simulink model "ADC"  (R2015a)
settings: Solver=ode4  StartTime=t0  StopTime=tf  FixedStep=dt  RelTol=1e-6
InitFcn:
  | sat_model_init
undefined symbols (not defined in the file or in its folder): Continuous, Time
libraries: simulink x1, ctrlSharedLib x1, dspmathops x1
settings Model: SimulationMode=external  Creator=Josue  LastModifiedBy=jbparham
settings DataIOCC: SignalLoggingSaveFormat=ModelDataLogs  SaveOutput=off  SaveState=on  SaveTime=off
settings OptimizationCC: ExpressionDepthLimit=2147483647  EfficientMapNaN2IntZero=off  OptimizeModelRefInitCode=on  LifeSpan=Inf
settings DebuggingCC: ReadBeforeWriteMsg=DisableAll  WriteAfterWriteMsg=DisableAll  WriteAfterReadMsg=DisableAll  UnderspecifiedInitializationDetection=Classic  MergeDetectMultiDrivingBlocksExec=none  SolverPrmCheckMsg=warning  MultiTaskDSMMsg=warning  MultiTaskCondExecSysMsg=none  FcnCallInpInsideContextMsg=UseLocalSettings  StateNameClashWarn=warning
settings HardwareCC: TargetBitPerLong=64  TargetBitPerPointer=64  TargetLongLongMode=on  TargetIntDivRoundTo=Zero  TargetEndianess=LittleEndian  TargetWordSize=64  TargetHWDeviceType=MATLAB Host  ProdEqTarget=off
settings ModelReferenceCC: ModelReferenceNumInstancesAllowed=Single
settings SFSimCC: SimParseCustomCode=off
settings RTWCC: SystemTargetFile=ert.tlc  TemplateMakefile=ert_default_tmf  Description=Embedded Coder  GenerateReport=on  IncludeHyperlinkInReport=on  LaunchReport=on
settings CodeAppCC: IgnoreCustomStorageClasses=off  MaxIdLength=128
settings ERTTargetCC: ParMdlRefBuildCompliant=on  CompOptLevelCompliant=on  ConcurrentExecutionCompliant=on  ERTFirstTimeCompliant=on  ModelStepFunctionPrototypeControlCompliant=on  CPPClassGenCompliant=on  InlinedParameterPlacement=Hierarchical  ERTCustomFileTemplate=example_file_process.tlc

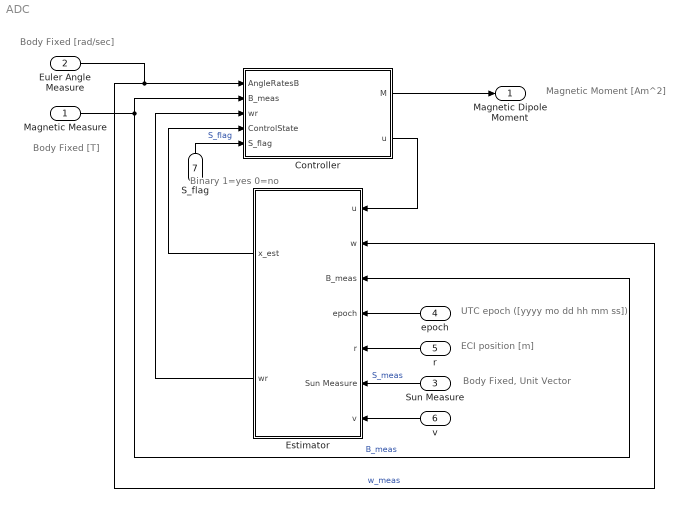
== system ADC ==
  note: Magnetic Moment [Am^2]
  note: Binary 1=yes 0=no
  note: ECI position [m]
  note: UTC epoch ([yyyy mo dd hh mm ss])
  note: Body Fixed, Unit Vector
  note: Body Fixed [rad/sec]
  note: Body Fixed [T]
  Magnetic Measure : Inport  OutDataTypeStr=double  PortDimensions=3  SampleTime=0
  Euler Angle Measure : Inport  Port=2  OutDataTypeStr=double  PortDimensions=3  SampleTime=0
  Sun Measure : Inport  Port=3  OutDataTypeStr=double  PortDimensions=3  SampleTime=0
  epoch : Inport  Port=4  OutDataTypeStr=double  PortDimensions=6
  r : Inport  Port=5  OutDataTypeStr=double  PortDimensions=3  SampleTime=0
  "v " : Inport  Port=6  OutDataTypeStr=double  PortDimensions=3  SampleTime=0
  S_flag : Inport  Port=7  OutDataTypeStr=double  PortDimensions=1  SampleTime=0
  Controller : Subsystem
  Estimator : Subsystem
  Magnetic Dipole Moment : Outport  OutDataTypeStr=double  PortDimensions=3  SampleTime=0
  wires:
  Magnetic Measure/1 -> Estimator/3(B_meas), Controller/2(B_meas)  "B_meas"
  Euler Angle Measure/1 -> Controller/1(AngleRatesB), Estimator/2(w)  "w_meas"
  Controller/1(M) -> Magnetic Dipole Moment/1
  Controller/2(u) -> Estimator/1(u)
  epoch/1 -> Estimator/4(epoch)
  r/1 -> Estimator/5(r)
  Sun Measure/1 -> Estimator/6(Sun Measure)  "S_meas"
  "v "/1 -> Estimator/7("v ")
  Estimator/1(x_est) -> Controller/4(ControlState)
  S_flag/1 -> Controller/5(S_flag)  "S_flag"
  Estimator/2(wr) -> Controller/3(wr)

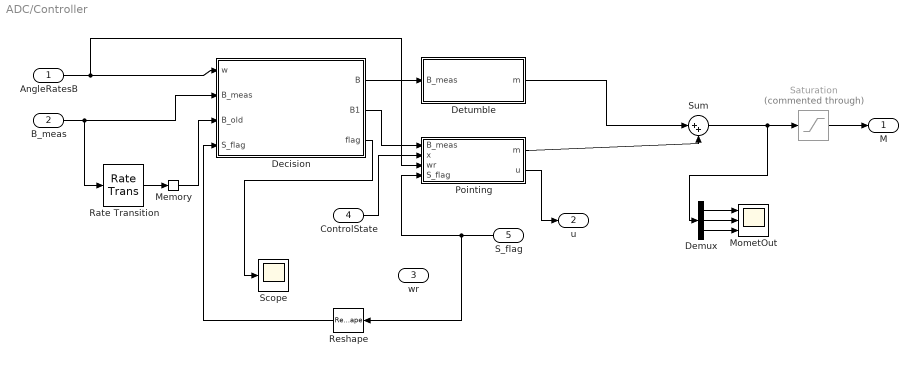
== system ADC/Controller ==
  AngleRatesB : Inport
  B_meas : Inport  Port=2
  wr : Inport  Port=3
  ControlState : Inport  Port=4
  S_flag : Inport  Port=5
  Decision : MATLAB Function  TreatAsAtomicUnit=on
  Demux : Demux  Outputs=3
  "Detumble " : Subsystem
  Memory : Memory  InheritSampleTime=on
  MometOut : Scope  NumInputPorts=3
      settings: YMin=-0.008~-0.015~-0.008  YMax=0.004~0.0175~0.002
  Pointing : Subsystem
  Rate Transition : RateTransition  OutPortSampleTime=.1
  Reshape : Reshape  OutputDimensionality=Customize
  Saturation : Saturate  Commented=through  UpperLimit=1  LowerLimit=-1
  Scope : Scope
      settings: YMin=0.95  YMax=1.05  SaveName=ScopeData5
  Sum : Sum  Inputs=|++
  M : Outport
  u : Outport  Port=2
  wires:
  Rate Transition/1 -> Memory/1
  S_flag/1 -> Reshape/1, Pointing/4(S_flag)
  Reshape/1 -> Decision/4(S_flag)
  B_meas/1 -> Decision/2(B_meas), Rate Transition/1
  Pointing/1(m) -> Sum/2
  Saturation/1 -> M/1
  Decision/3(flag) -> Scope/1
  Memory/1 -> Decision/3(B_old)
  Demux/3 -> MometOut/3
  Demux/2 -> MometOut/2
  Demux/1 -> MometOut/1
  Pointing/2(u) -> u/1
  ControlState/1 -> Pointing/2(x)
  Decision/2(B1) -> Pointing/1(B_meas)
  Decision/1(B) -> "Detumble "/1("B_meas ")
  "Detumble "/1(m) -> Sum/1
  Sum/1 -> Saturation/1, Demux/1
  AngleRatesB/1 -> Decision/1(w), Pointing/3(wr)

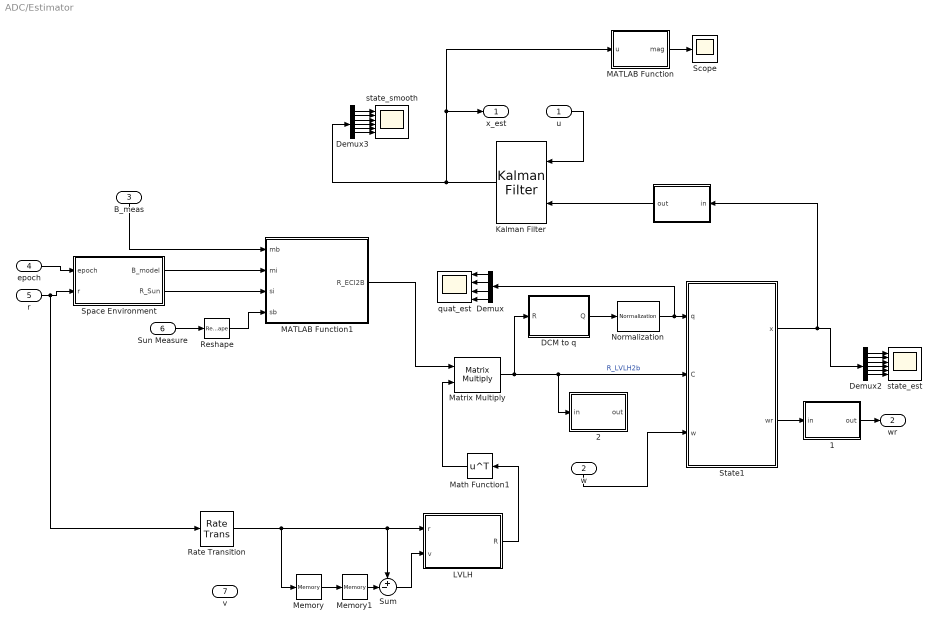
== system ADC/Estimator ==
  u : Inport
  w : Inport  Port=2
  B_meas : Inport  Port=3
  epoch : Inport  Port=4
  r : Inport  Port=5
  Sun Measure : Inport  Port=6
  "v " : Inport  Port=7
  " " : MATLAB Function  TreatAsAtomicUnit=on
  " 1" : MATLAB Function  TreatAsAtomicUnit=on
  " 2" : MATLAB Function  TreatAsAtomicUnit=on
  " LVLH " : MATLAB Function  TreatAsAtomicUnit=on
  DCM to q : MATLAB Function  TreatAsAtomicUnit=on
  Demux : Demux
  Demux2 : Demux  Outputs=6
  Demux3 : Demux  Outputs=6
  Kalman Filter : ctrlSharedLib/Kalman Filter  TimeDomain=Continuous-Time  UseCurrentEstimator=on  ModelSource=Individual A, B, C, D matrices  ModelSourceVariable=ss(0.95,1,1,0,1)  A=[0,0,0,1,0,0;0,0,0,0,1,0;0,0,0,0,0,1;3.26658658709613e-06,0,0,0,0,0.00184463935812897;0,2.93992792838652e-06,0,0,0,0;0,0,-3.49991420046014e-07,-0.000790559724912417,0,0]  B=[zeros(3);eye(3)]  C=eye(6)  D=0  NumberOfStates=1  NumberOfInputs=1  NumberOfOutputs=1  InitialEstimateSource=Dialog  X0=zeros(6,1)  P0=10  UseK=off  UseGH=off  NumberOfProcessNoiseInputs=1  G=1  TimeInvariantG=on  H=0  TimeInvariantH=on  Q=1  TimeInvariantQ=on  R=[.5*eye(3),zeros(3);zeros(3),0.005*eye(3)]  TimeInvariantR=on  N=0  TimeInvariantN=on  AddInputPort=on  AddEnablePort=off  ExternalReset=none  OutputEstimatedY=off  OutputP=off  Ts=.1
  MATLAB Function : MATLAB Function  TreatAsAtomicUnit=on
  MATLAB Function1 : MATLAB Function  TreatAsAtomicUnit=on
  Math Function1 : Math  Operator=transpose  SaturateOnIntegerOverflow=on
  Matrix Multiply : Product  Multiplication=Matrix(*)
  Memory : Memory
  Memory1 : Memory
  Normalization : dspmathops/Normalization  NormType=Squared 2-norm  Bias=1e-10  NormOver=Each column  ColComp=off  Dimension=1  outputDataTypeStr=Inherit: Same as product output  outputLastDataTypeStr=Inherit: Same as product output  outputMin=[]  outputMax=[]  accumDataTypeStr=Inherit: Same as product output  accumLastDataTypeStr=Inherit: Same as product output  roundingMode=Floor  overflowMode=off
  Rate Transition : RateTransition  OutPortSampleTime=.1
  Reshape : Reshape  OutputDimensionality=Customize  OutputDimensions=[3,1]
  Scope : Scope
      settings: YMin=5.55112e-17  YMax=1.4  SaveName=ScopeData3
  Space Environment : Subsystem
  State1 : MATLAB Function  TreatAsAtomicUnit=on
  Sum : Sum  Inputs=+-|
  quat_est : Scope  NumInputPorts=4
      settings: ShowLegends=on  YMin=-1.24924~-1.24976~-1.2264~-0.115999  YMax=1.24823~1.24976~1.22612~1.04399  SaveName=quat_est  DataFormat=Structure
  state_est : Scope  NumInputPorts=6
      settings: ShowLegends=on  YMin=-1.23534~-1.22576~-1.24248~-0.102409~-0.112864~-0.0966162  YMax=1.24677~1.22585~1.24228~0.115625~0.0969559~0.105  SaveName=quat_est1  DataFormat=Structure
  state_smooth : Scope  NumInputPorts=6
      settings: ShowLegends=on  YMin=-1~-1~-1~-0.075~-0.1~-0.075  YMax=1~1~1~0.1~0.075~0.1  SaveName=ScopeData4  DataFormat=Structure
  x_est : Outport
  wr : Outport  Port=2
  wires:
  Rate Transition/1 -> Memory/1, Sum/1, " LVLH "/1(r)
  Sum/1 -> " LVLH "/2(v)
  Memory1/1 -> Sum/2
  Memory/1 -> Memory1/1
  Reshape/1 -> MATLAB Function1/4(sb)
  Sun Measure/1 -> Reshape/1
  Kalman Filter/1 -> x_est/1, MATLAB Function/1(u), Demux3/1
  " "/1(out) -> Kalman Filter/2
  u/1 -> Kalman Filter/1
  Demux3/6 -> state_smooth/6
  Demux3/5 -> state_smooth/5
  Demux3/3 -> state_smooth/3
  Demux3/4 -> state_smooth/4
  Demux3/2 -> state_smooth/2
  Demux3/1 -> state_smooth/1
  " 1"/1(out) -> wr/1
  State1/2(wr) -> " 1"/1(in)
  Demux2/6 -> state_est/6
  Demux2/5 -> state_est/5
  Demux2/3 -> state_est/3
  Demux2/4 -> state_est/4
  Demux2/2 -> state_est/2
  Demux2/1 -> state_est/1
  State1/1(x) -> Demux2/1, " "/1(in)
  B_meas/1 -> MATLAB Function1/1(mb)
  w/1 -> State1/3(w)
  MATLAB Function1/1(R_ECI2B) -> Matrix Multiply/1
  Space Environment/1(B_model) -> MATLAB Function1/2(mi)
  MATLAB Function/1(mag) -> Scope/1
  Normalization/1 -> State1/1(q), Demux/1
  Space Environment/2(R_Sun) -> MATLAB Function1/3(si)
  Demux/3 -> quat_est/3
  Matrix Multiply/1 -> DCM to q/1(R), State1/2(C), " 2"/1(in)  "R_LVLH2b"
  Demux/4 -> quat_est/4
  Demux/2 -> quat_est/2
  epoch/1 -> Space Environment/1(epoch)
  r/1 -> Rate Transition/1, Space Environment/2(r)
  DCM to q/1(Q) -> Normalization/1
  Demux/1 -> quat_est/1
  Math Function1/1 -> Matrix Multiply/2
  " LVLH "/1(R) -> Math Function1/1

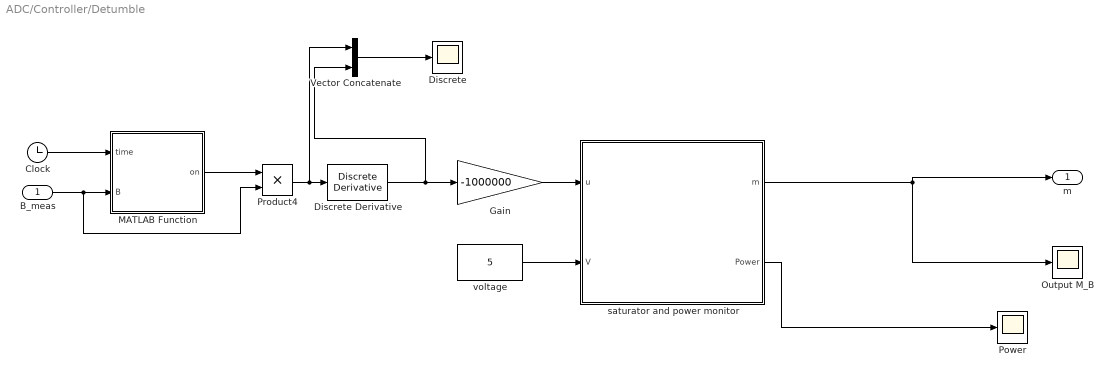
== system ADC/Controller/Detumble  ==
  "B_meas " : Inport
  Clock : Clock
  "Discrete " : Scope
      settings: ShowLegends=on  TimeRange=0.0243621865078012  YMin=-5.004965470144639e-05  YMax=3.166418994305964e-05  SaveName=ScopeData2
  Discrete Derivative : simulink/Discrete/Discrete Derivative  gainval=1.0  ICPrevScaledInput=0  InputProcessing=Inherited  OutMin=[]  OutMax=[]  OutDataType=fixdt(1, 16)  OutScaling=2^-10  DoSatur=off
  Gain : Gain  Gain=-1000000
  MATLAB Function : MATLAB Function  TreatAsAtomicUnit=on
  Output M_B : Scope
      settings: TimeRange=100000  YMin=-3  YMax=3
  Power : Scope
      settings: TimeRange=693.5918147549814  YMin=0.1  YMax=2.4  SaveName=Power_Data
  Product4 : Product
  Vector Concatenate : Concatenate
  saturator and power monitor : MATLAB Function  TreatAsAtomicUnit=on
  voltage : Constant  Value=5
  m : Outport
  wires:
  Vector Concatenate/1 -> "Discrete "/1
  Product4/1 -> Discrete Derivative/1, Vector Concatenate/1
  Gain/1 -> saturator and power monitor/1(u)
  Discrete Derivative/1 -> Gain/1, Vector Concatenate/2
  "B_meas "/1 -> MATLAB Function/2(B), Product4/2
  MATLAB Function/1(on) -> Product4/1
  Clock/1 -> MATLAB Function/1(time)
  saturator and power monitor/2(Power) -> Power/1
  voltage/1 -> saturator and power monitor/2(V)
  saturator and power monitor/1(m) -> m/1, Output M_B/1

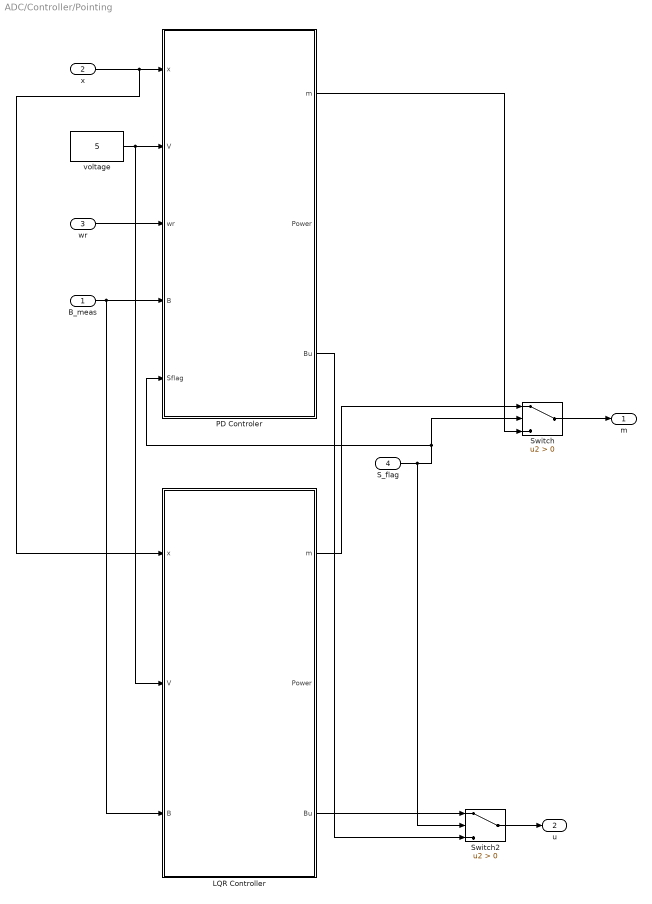
== system ADC/Controller/Pointing ==
  B_meas : Inport
  x : Inport  Port=2
  wr : Inport  Port=3
  S_flag : Inport  Port=4
  LQR Controller : MATLAB Function  TreatAsAtomicUnit=on
  PD Controler : MATLAB Function  TreatAsAtomicUnit=on
  Switch : Switch  Criteria=u2 > Threshold
  Switch2 : Switch  Criteria=u2 > Threshold
  voltage : Constant  Value=5
  m : Outport
  u : Outport  Port=2
  wires:
  PD Controler/3(Bu) -> Switch2/3
  Switch2/1 -> u/1
  LQR Controller/3(Bu) -> Switch2/1
  LQR Controller/1(m) -> Switch/1
  PD Controler/1(m) -> Switch/3
  B_meas/1 -> PD Controler/4(B), LQR Controller/3(B)
  S_flag/1 -> PD Controler/5(Sflag), Switch/2, Switch2/2
  Switch/1 -> m/1
  wr/1 -> PD Controler/3(wr)
  x/1 -> PD Controler/1(x), LQR Controller/1(x)
  voltage/1 -> PD Controler/2(V), LQR Controller/2(V)

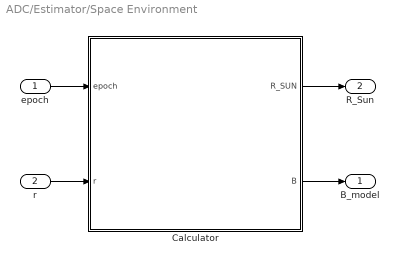
== system ADC/Estimator/Space Environment ==
  epoch : Inport
  r : Inport  Port=2
  Calculator : MATLAB Function  TreatAsAtomicUnit=on
  B_model : Outport
  R_Sun : Outport  Port=2
  wires:
  Calculator/2(B) -> B_model/1
  r/1 -> Calculator/2(r)
  epoch/1 -> Calculator/1(epoch)
  Calculator/1(R_SUN) -> R_Sun/1

== matlab function ADC/Controller/Decision ==
  data: w input; B output; B_meas input; B1 output; B_old input; flag output; S_flag input
function [B,B1,flag] = det_or_point(w,B_meas,B_old,S_flag)
%B is output to Detumbler, B1 is output to Pointing Control
flag=0;
if (abs(norm(w)) >= 0.01) || (norm(B_meas-B_old)/norm(B_meas)>0.05 )
    B = B_meas;
    B1 = [0;0;0];
else
    B = [0;0;0];
    B1 = B_meas;
    flag=1;
end

end

== matlab function ADC/Controller/Detumble /saturator and power monitor ==
  data: u input; m output; V input; Power output
function [m,Power] = coil(u,V)


I_max=[.08;.08;.08];
m_max = [.2;.2;.2];

m=[0;0;0];
m_raw=u;

%Saturator
if abs(m_raw(1))>m_max(1)
    m(1)=m_max(1)*sign(m_raw(1));
else
    m(1)=m_raw(1);
end

if abs(m_raw(2))>m_max(2)
    m(2)=m_max(2)*sign(m_raw(2));
else
    m(2)=m_raw(2);
end

if abs(m_raw(3))>m_max(3)
    m(3)=m_max(3)*sign(m_raw(3));
else
    m(3)=m_raw(3);
end
%Power Monitor
I_tot=abs(I_max(1)*m(1)/m_max(1))+abs(I_max(2)*m(2)/m_max(2))+abs(I_max(3)*m(3)/m_max(3));
Power=V*I_tot;
end

== matlab function ADC/Controller/Pointing/LQR Controller ==
  data: x input; m output; V input; Power output; B input; Bu output
function [m,Power,Bu] = coil(x,V,B)
%maximum magnetic moment
I_max=[.08;.08;.08];
m_max=[.2;.2;.2];
m=[0;0;0];

% Main Controller
K=[1015.81637123020,8.04611892244142e-14,-453.958044168676,384003.046505704,1.44940442674718e-11,-187075.587093135;7.60272150440681e-14,1186.23970592244,-2.35978593865247e-13,1.08705332006039e-11,448289.486640409,9.49012273578315e-11;453.958044168675,-1.67413778929006e-14,600.766687834337,-20043.8129028358,1.35573181939759e-11,795987.850800695];
m_raw=-skew(B)*K*x;
u=-K*x;
Bu=[1.57407015004541e-08,0,0;0,1.18055261253406e-08,0;0,0,1.68650373219151e-09]*u;

%Saturator
if abs(m_raw(1))>m_max(1)
    m(1)=m_max(1)*sign(m_raw(1));
else
    m(1)=m_raw(1);
end

if abs(m_raw(2))>m_max(2)
    m(2)=m_max(2)*sign(m_raw(2));
else
    m(2)=m_raw(2);
end

if abs(m_raw(3))>m_max(3)
    m(3)=m_max(3)*sign(m_raw(3));
else
    m(3)=m_raw(3);
end
%Power Monitor
I_tot=abs(I_max(1)*m(1)/m_max(1))+abs(I_max(2)*m(2)/m_max(2))+abs(I_max(3)*m(3)/m_max(3));
Power=V*I_tot;

end

function A = skew(x)

A = [0    -x(3)  x(2);
     x(3)  0    -x(1);
    -x(2)  x(1)  0];
 
end

== matlab function ADC/Estimator/Space Environment/Calculator ==
  data: epoch input; r input; R_SUN output; B output
function [R_SUN,B] =space_env(epoch,r)

Re = 6378.1363e3;
%Compute the Julian Date (JD) from a Gregorian Date (UT1) input
yr=epoch(1);  %(year)
mo=epoch(2);  %(month)
d=epoch(3);  %(day)
h=epoch(4);  %(hr)
min=epoch(5);  %(min)
s=epoch(6);  %(sec)
JD=367*yr-floor(7/4*(yr+floor((mo+9)/12)))+floor(275*mo/9)+d+1721013.5+(((s/60+min)/60)+h)/24;  %(JD)

%Compute the Universal Time (UT) from JD
T_UT1 = (JD-2451545.0)/36525;

%Compute the Greenwich Mean Sidereal Time (GMST) from UT
GMST = 67310.54841 + (876600.0*3600.0 + 8640184.812866)*T_UT1 + 0.093104*T_UT1^2 - 6.2E-6*T_UT1^3;
G0 = rem(GMST,86400)/240;
if G0 < 0
    G0 = -(-G0-360);
end
%truncate GMST between 0 and 2pi
GMST = G0*pi/180;  %(rad)

%Compute the Direction Cosine Matrix (DCM) for converting vectors in 
%Earth-Centered Inertial (ECI) frame to vectors in Earth-Centered 
%Earth-Fixed (ECEF) frame
R_ECItoECEF = ROT3(GMST);

%Compute the Sun vector based on the UT
R_SUN = r_sun(T_UT1);

%Compute the Moon vector based on the UT
R_MOON = r_moon(T_UT1,Re);

%Compute the Earth's magnetic vector in the ECI frame
B = Dipole_model(r,GMST,Re);  %(T)

end

function A = ROT3(theta)

A = [cos(theta) sin(theta) 0;
    -sin(theta) cos(theta) 0;
     0          0          1];
 
end

function r = r_sun(T_UT1)

lambdaM = 280.4606184+36000.77005361*T_UT1;  %(°)
M = (357.5277233+35999.05034*T_UT1)*pi/180.0;  %(rad)
lambdaecliptic = (lambdaM+1.914666471*sin(M)+0.019994643*sin(2*M))*pi/180.0;  %(rad)
E = (23.439291-0.0130042*T_UT1)*pi/180.0;  %(rad)
Rs = (1.000140612-0.016708617*cos(M)-0.000139589*cos(2*M))*149598000*10^3;  %(m)
r = Rs*[cos(lambdaecliptic);
        cos(E)*sin(lambdaecliptic);
        sin(E)*sin(lambdaecliptic)];  %(m)
  
end

function r = r_moon(T_UT1,Re)

lambdaecliptic = (218.32+481267.8813*T_UT1+6.29*sin((134.9+477198.85*T_UT1)*pi/180)-...
                 1.27*sin((259.2-413335.38*T_UT1)*pi/180)+0.66*sin((235.7+890534.23*T_UT1)*pi/180)+...
                 0.21*sin((269.9+954397.70*T_UT1)*pi/180)-0.19*sin((357.5+35999.05*T_UT1)*pi/180)-...
                 0.11*sin((186.6+966404.05*T_UT1)*pi/180))*pi/180;  %(rad)
phiecliptic = (5.13*sin((93.3+483202.03*T_UT1)*pi/180)+0.28*sin((228.2+960400.87*T_UT1)*pi/180)-...
              0.28*sin((318.3+6003.18*T_UT1)*pi/180)-0.17*sin((217.6-407332.20*T_UT1)*pi/180))*pi/180;  %(rad)
P = (0.9508+0.0518*cos((134.9+477198.85*T_UT1)*pi/180)+0.0095*cos((259.2-413335.38*T_UT1)*pi/180)+...
    0.0078*cos((235.7+890534.23*T_UT1)*pi/180)+0.0028*cos((269.9+954397.70*T_UT1)*pi/180))*pi/180;  %(rad)
epsilon = (23.439291-0.0130042*T_UT1-1.64E-7*T_UT1^2+5.04E-7*T_UT1^3)*pi/180; %rad
radius = Re/sin(P);  %(m)
r = radius*[cos(phiecliptic)*cos(lambdaecliptic);
            cos(epsilon)*cos(phiecliptic)*sin(lambdaecliptic)-sin(epsilon)*sin(phiecliptic);
            sin(epsilon)*cos(phiecliptic)*sin(lambdaecliptic)+cos(epsilon)*sin(phiecliptic)];  %(m)
        
end

function B = Dipole_model(r,GMST,Re)

%2010 IGRF constants
g01 = -29496.5e-9;
g11 = -1585.9e-9;
h11 = 4945.1e-9;

H0 = sqrt(g01^2 + g11^2 + h11^2);

theta_m = acos(g01/H0);
phi_m = atan2(h11,g11);

GMST_m = GMST + phi_m;

m_hat = [sin(theta_m)*cos(GMST_m);
         sin(theta_m)*sin(GMST_m);
         cos(theta_m)];
     
r_hat = r/norm(r);
     
B = Re^3*H0/norm(r)^3*(3*dot(m_hat,r_hat)*r_hat - m_hat);

end

== matlab function ADC/Controller/Detumble /MATLAB Function ==
  data: time input; on output; B input
function on = clock_timer(time,B)
persistent counter
persistent times

time_diff=1;
if isempty(times)
    times = zeros(1,1000000);
end
if isempty(counter)
    counter = 1;
end
if(norm(B)>0)
    times(1,counter)=time;
    if(counter>1)
        time_diff=times(1,counter)-times(1,(counter-1));
    end
    if(time_diff>=1)
        on=0;
    else
        on=1;
        
%         counter=1;
        if(counter==1000000)
            counter=1;
            times=zeros(1,1000000);
        end
    end
    
    counter=counter+1;
else
    on=0;
end  
    
end

== matlab function ADC/Estimator/DCM to q ==
  data: R input; Q output
function Q = DCM_to_q(R)
%#codegen
q=zeros(4,1);

q(4)=0.5*sqrt(max(trace(R),-1)+1);
q(1)=(R(2,3)-R(3,2))/(4*q(4));
q(2)=(R(3,1)-R(1,3))/(4*q(4));
q(3)=(R(1,2)-R(2,1))/(4*q(4));

Q=q;

== matlab function ADC/Controller/Pointing/PD Controler ==
  data: x input; m output; V input; wr input; Power output; B input; Bu output; Sflag input
function [m,Power,Bu] = coil_pd(x,V,wr,B,Sflag)
%maximum magnetic moment
I_max=[.08;.08;.08];
m_max=[.2;.2;.2];
m=[0;0;0];

%Full Mule
Jx=0.06;
Jy=0.1;
Jz=0.14;
J = [Jx  0  0;
      0  Jy 0;
      0  0  Jz];  %centroidal moment of inertia sans reaction wheel system (kg-m^2)

wr=wr+[0;0.0011;0];

% Main PID Controller
dq=x(1:3,:);
Omega=skew(wr);
wn=0.0011*2;
xi=sqrt(2)/2;
D=2*xi*wn*J;
K=2*wn^2*J;

% from Wie et. al
u= - Omega*J*wr - D*wr - 0*K*dq;

if norm(B)>0
    m_raw= cross(B,u)/norm(B)^2;
else
    m_raw=zeros(3,1);
end

%Saturator
if abs(m_raw(1))>m_max(1)
    m(1)=m_max(1)*sign(m_raw(1));
else
    m(1)=m_raw(1);
end

if abs(m_raw(2))>m_max(2)
    m(2)=m_max(2)*sign(m_raw(2));
else
    m(2)=m_raw(2);
end

if abs(m_raw(3))>m_max(3)
    m(3)=m_max(3)*sign(m_raw(3));
else
    m(3)=m_raw(3);
end
%Power Monitor
I_tot=abs(I_max(1)*m(1)/m_max(1))+abs(I_max(2)*m(2)/m_max(2))+abs(I_max(3)*m(3)/m_max(3));
Power=V*I_tot;

% control torque
Bu=cross(m,B);

end

function A = skew(x)

A = [0    -x(3)  x(2);
     x(3)  0    -x(1);
    -x(2)  x(1)  0];
 
end

== matlab function ADC/Estimator/State1 ==
  data: x output; q input; C input; w input; wr output
function [x,wr]  = qw2state(q,C,w)
%#codegen
% w_r=w+.0011*R(:,2);
% q_dot=0.5*[q(4) -q(3)  q(2)
%        q(3)  q(4) -q(1)
%        -q(2) q(1)  q(4)]*w_r;

% orbital rate in rad/sec = 0.0011
wr=w+C(:,2)*0.0011;
q_dot =quat_EOM(wr,q);
    
q_otob=[q(1);q(2);q(3)];
x=[q_otob; q_dot(1:3)];

end

function q_BtoECI_dot = quat_EOM(w_BwrtECI_B,q_BtoECI)
% This block supports an embeddable subset of the MATLAB language.
% See the help menu for details. 

q_BtoECI_dot = 1/2*Xi_matrix(q_BtoECI)*w_BwrtECI_B;
          
end

function A = Xi_matrix(q)

A = [q(4,1)*eye(3)+skew(q(1:3,1));
    -q(1:3,1)'];
 
end

function A = skew(x)

A = [0    -x(3)  x(2);
     x(3)  0    -x(1);
    -x(2)  x(1)  0];
 
end

== matlab function ADC/Estimator/ LVLH  ==
  data: r input; R output; v input
function R = R_inertial2lvlh(r,v)
%% create Local Horizontal Local Vertical Coordinates
%#codegen
z=-unit(r);

if norm(v)>1e-8
    % use this if reasonable velocity estimate from postion change
    x=unit(v-dot(v,z)*z);
    y=cross(z,x);
else
    % assume polar and use geometry to find velocity direction
    y_tmp=unit([[0,-1;1,0]*[r(1);r(2)];0]);
    y=unit(y_tmp-dot(y_tmp,z)*z);
    x=cross(y,z);
end

R=[x';y';z'];
end

function a = unit(A)
a = A/norm(A);
end

== matlab function ADC/Estimator/MATLAB Function ==
  data: u input; mag output
function mag  = norm_scope(u)
%#codegen
mag=norm(u);

== matlab function ADC/Estimator/MATLAB Function1 ==
  data: mb input; mi input; R_ECI2B output; si input; sb input
function R_ECI2B = TRIAD(mb,mi,si,sb)

W1 = mb/norm(mb);
W2 = sb/norm(sb);
V1 = mi/norm(mi);
V2 = si/norm(si);

r1=V1;
r2=cross(V1,V2)/norm(cross(V1,V2));
r3=cross(V1,cross(V1,V2))/norm(cross(V1,V2));

s1=W1;
s2=cross(W1,W2)/norm(cross(W1,W2));
s3=cross(W1,cross(W1,W2))/norm(cross(W1,W2));

R_ECI2B=s1*r1'+ s2*r2' + s3*r3';

== matlab function ADC/Estimator/  ==
  data: in input; out output
function out  = check_data(in)
%#codegen
in(isnan(in))=0;
out=in;

== matlab function ADC/Estimator/ 1 ==
  data: in input; out output
function out  = check_data(in)
%#codegen
in(isnan(in))=0;
out=in;

== matlab function ADC/Estimator/ 2 ==
  data: in input; out output
function out  = check_data(in)
%#codegen
if isnan(sum(sum([nan 0 0; 0 0 0; 0 0 0])))>0
    out = eye(3);
else
    out = in;
end
